simulink model "SMC_TwoLink_Inverse"  (R2020b)
settings: Solver=VariableStepAuto  StartTime=0.0  StopTime=10.0  MaxStep=0.0005  RelTol=1e-3
settings Model: Creator=MR.co  LastModifiedBy=MR.co

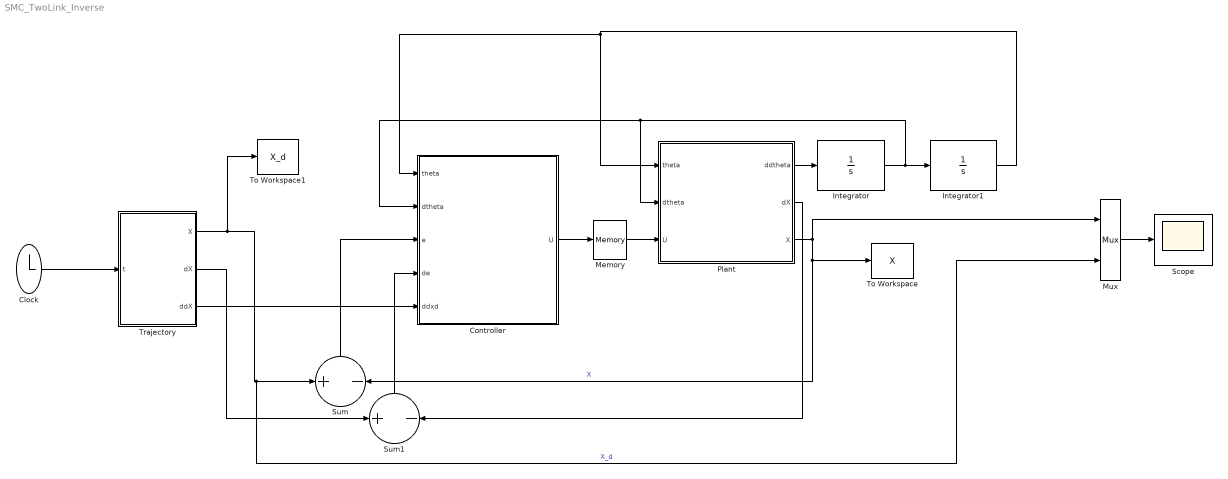
== system SMC_TwoLink_Inverse ==
  Clock : Clock
  Controller : MATLAB Function  TreatAsAtomicUnit=on
  Integrator : Integrator  InitialCondition=randn(2,1)
  Integrator1 : Integrator  InitialCondition=randn(2,1)
  Memory : Memory
  Mux : Mux  Inputs=2
  Plant : MATLAB Function  TreatAsAtomicUnit=on
  Scope : Scope
  Sum : Sum  Inputs=+|-
  Sum1 : Sum  Inputs=+|-
  To Workspace : ToWorkspace  VariableName=X  SampleTime=-1
      settings: Save2DSignal=2-D array (concatenate along first dimension)
  To Workspace1 : ToWorkspace  VariableName=X_d  SampleTime=-1
      settings: Save2DSignal=2-D array (concatenate along first dimension)
  Trajectory : MATLAB Function  TreatAsAtomicUnit=on
  wires:
  Controller/1(U) -> Memory/1
  Plant/1(ddtheta) -> Integrator/1
  Integrator1/1 -> Controller/1(theta), Plant/1(theta)
  Integrator/1 -> Plant/2(dtheta), Controller/2(dtheta), Integrator1/1
  Clock/1 -> Trajectory/1(t)
  Trajectory/3(ddX) -> Controller/5(ddxd)
  Plant/3(X) -> Sum/2, To Workspace/1, Mux/1  "X"
  Trajectory/1(X) -> To Workspace1/1, Mux/2, Sum/1  "X_d"
  Sum/1 -> Controller/3(e)
  Plant/2(dX) -> Sum1/2
  Sum1/1 -> Controller/4(de)
  Mux/1 -> Scope/1
  Trajectory/2(dX) -> Sum1/1
  Memory/1 -> Plant/3(U)

== matlab function SMC_TwoLink_Inverse/Controller ==
  data: theta input; U output; dtheta input; e input; de input; ddxd input
function U = fcn(theta , dtheta , e  , de , ddxd)

    L1 = 1; % m
    L2 = 1.2; % m
    
    Lc1 = .5; % m
    Lc2 = .6; % m
     
    m1 = 1; % Kg
    m2 = 2; % Kg
    
    I1 = 1/12 * m1 * L1^2;  %kg.N
    I2 = 1/12 * m2 * L2^2;  %kg.N

    g = 9.8; % m/s^2
   
    
    M11 = m1 * Lc1^2 + I1 + m2*(L1^2 + Lc2^2 + 2 * L1 * Lc2 * cos(theta(2))) + I2;
    M12 = m2 * L1 * Lc2 * cos(theta(2)) + m2 * Lc2^2 + I2;
    M22 = m2 * Lc2^2 + I2;
    M=[M11 M12;M12 M22];

    G1 = m1 * Lc1 * cos(theta(1)) + m2 * (Lc2 * cos(theta(1) + theta(2)) + L1 * cos(theta(1)));
    G2 = m2 * Lc2 * cos(theta(1) + theta(2));
    G=[G1*g;G2*g];
    
    F12 = m2 * L1 * Lc2 * sin(theta(2));
    C=[-F12*dtheta(2) -F12*(dtheta(1)+dtheta(2));F12*dtheta(1) 0];
    

    J11 = -L1 * sin(theta(1)) - L2 * sin(theta(1) + theta(2));
    J12 = -L2 * sin(theta(1) + theta(2)) ;


    J21 = L1 * cos(theta(1)) + L2 * cos(theta(1) + theta(2));
    J22 = L2 * cos(theta(1) + theta(2)) ;

    J = [J11 J12; J21 J22];


    dJ11 = -L1 * cos(theta(1))*(dtheta(1)) - L2 * cos(theta(1) + theta(2))*(dtheta(1)+dtheta(2)) ;
    dJ12 = -L2 * cos(theta(1) + theta(2))*(dtheta(1)+dtheta(2));


    dJ21 = -L1 * sin(theta(1))*(dtheta(1)) - L2 * sin(theta(1) + theta(2))*(dtheta(1)+dtheta(2)) ;
    dJ22 = -L2 * sin(theta(1) + theta(2))*(dtheta(1)+dtheta(2));


    dJ = [dJ11 dJ12 ; dJ21 dJ22 ];
    
    c = 10 * eye(2);
    ebs = 10 * eye(2);
    
    s = de + c*e;
    
    V = J\(ddxd + c*de + ebs * sign(s) - dJ*dtheta);

    U = M * V + C*dtheta + G;

== matlab function SMC_TwoLink_Inverse/Plant ==
  data: theta input; ddtheta output; dtheta input; U input; dX output; X output
function [ddtheta , dX , X] = fcn(theta , dtheta ,U)

    L1 = 1; % m
    L2 = 1.2; % m
    
    Lc1 = .5; % m
    Lc2 = .6; % m
     
    m1 = 1; % Kg
    m2 = 2; % Kg
    
    I1 = 1/12 * m1 * L1^2;  %kg.N
    I2 = 1/12 * m2 * L2^2;  %kg.N

    g = 9.8; % m/s^2
   
    
    M11 = m1 * Lc1^2 + I1 + m2*(L1^2 + Lc2^2 + 2 * L1 * Lc2 * cos(theta(2))) + I2;
    M12 = m2 * L1 * Lc2 * cos(theta(2)) + m2 * Lc2^2 + I2;
    M22 = m2 * Lc2^2 + I2;
    M=[M11 M12;M12 M22];

    G1 = m1 * Lc1 * cos(theta(1)) + m2 * (Lc2 * cos(theta(1) + theta(2)) + L1 * cos(theta(1)));
    G2 = m2 * Lc2 * cos(theta(1) + theta(2));
    G=[G1*g;G2*g];
    
    F12 = m2 * L1 * Lc2 * sin(theta(2));
    C=[-F12*dtheta(2) -F12*(dtheta(1)+dtheta(2));F12*dtheta(1) 0];
    
    
    ddtheta = M\( U -C*dtheta -G );

    J11 = -L1 * sin(theta(1)) - L2 * sin(theta(1) + theta(2));
    J12 = -L2 * sin(theta(1) + theta(2)) ;


    J21 = L1 * cos(theta(1)) + L2 * cos(theta(1) + theta(2));
    J22 = L2 * cos(theta(1) + theta(2)) ;

    J = [J11 J12; J21 J22];

% 
%     dJ11 = -L1 * cos(theta(1))*(dtheta(1)) - L2 * cos(theta(1) + theta(2))*(dtheta(1)+dtheta(2)) ;
%     dJ12 = -L2 * cos(theta(1) + theta(2))*(dtheta(1)+dtheta(2));
% 
% 
%     dJ21 = -L1 * sin(theta(1))*(dtheta(1)) - L2 * sin(theta(1) + theta(2))*(dtheta(1)+dtheta(2)) ;
%     dJ22 = -L2 * sin(theta(1) + theta(2))*(dtheta(1)+dtheta(2));
% 

%     dJ = [dJ11 dJ12 ; dJ21 dJ22 ];


    x = L1 * cos(theta(1)) + L2 * cos(theta(1)+theta(2));
    y = L1 * sin(theta(1)) + L2 * sin(theta(1)+theta(2));
    X = [x;y];

    dX = J * dtheta;

== matlab function SMC_TwoLink_Inverse/Trajectory ==
  data: t input; X output; dX output; ddX output
function [X , dX , ddX] = fcn(t)

 x = ((0.8+0.6* cos(pi*t)));
 y = ((1.2+0.6* sin(pi*t)));

 dx = -(3*pi*sin(pi*t))/5;
 dy = (3*pi*cos(pi*t))/5;

 ddx = -(3*pi^2*cos(pi*t))/5;
 ddy = -(3*pi^2*sin(pi*t))/5;

 
 X = [x;y];
 dX = [dx ; dy];
 ddX = [ddx ; ddy];
